simulink model "ex11"  (Simulink 6.0)
settings: Solver=VariableStepDiscrete  StartTime=0.0  StopTime=2  RelTol=1e-3
libraries: commutil2 x4, commsink2 x2, commdigbbndam2 x2, commfilt2 x2, dspsigops x2, commchan2 x1, commrandsrc2 x1
settings Model: LastModifiedBy=lxy

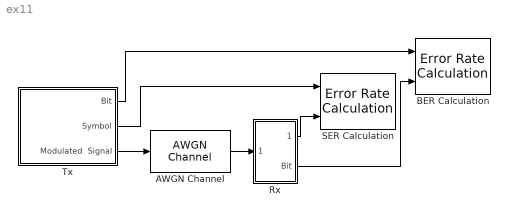
== system ex11 ==
  AWGN Channel : commchan2/AWGN Channel  seed=1234  noiseMode="Signal to noise ratio  (Es/No)"  EbNodB=10  EsNodB=SNR  SNRdB=10  bitsPerSym=1  Ps=0.5  Tsym=1/100000  variance=1
  BER Calculation : commsink2/Error Rate Calculation  N=0  st_delay=16  cp_mode=Entire frame  subframe=[]  PMode=Workspace  WsName=BER  RsMode2=off  stop=off  numErr=100  maxBits=1e6
  Rx : Subsystem
  SER Calculation : commsink2/Error Rate Calculation  N=0  st_delay=8  cp_mode=Entire frame  subframe=[]  PMode=Workspace  WsName=SER  RsMode2=off  stop=off  numErr=100  maxBits=1e6
  Tx : Subsystem
  wires:
  Tx/3(Modulated  Signal) -> AWGN Channel/1
  AWGN Channel/1 -> Rx/1(In1)
  Tx/2(Symbol) -> SER Calculation/1
  Rx/1(Symbol) -> SER Calculation/2
  Tx/1(Bit) -> BER Calculation/1
  Rx/2(Bit) -> BER Calculation/2

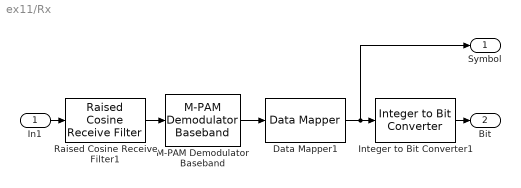
== system ex11/Rx ==
  In1 : Inport  Port=1  LatchInput=off
  Data Mapper1 : commutil2/Data Mapper  MapMode=Gray to Binary  M=4  MapVec=[0 1 3 2 7 6 4 5]
  Integer to Bit Converter1 : commutil2/Integer to Bit Converter  nbits=2
  M-PAM Demodulator Baseband : commdigbbndam2/M-PAM Demodulator Baseband  M=4  OutType=Integer  Dec=Binary  PowType=Min. distance between symbols  MinDist=2  AvgPow=1  PeakPow=1  numSamp=1
  Raised Cosine Receive Filter1 : commfilt2/Raised Cosine Receive Filter  filtType=Square root  N=10  D=4  R=0.25  sampMode=Frame-based  rateMode=Downsampling  downFactor=10  downOffset=0  checkGain=Normalized  filterGain=1  checkCoeff=off  variableName=rcRxFilt1  launchFVT=off
  Symbol : Outport
  Bit : Outport  Port=2
  wires:
  M-PAM Demodulator Baseband/1 -> Data Mapper1/1
  Integer to Bit Converter1/1 -> Bit/1
  Data Mapper1/1 -> Integer to Bit Converter1/1, Symbol/1
  In1/1 -> Raised Cosine Receive Filter1/1
  Raised Cosine Receive Filter1/1 -> M-PAM Demodulator Baseband/1

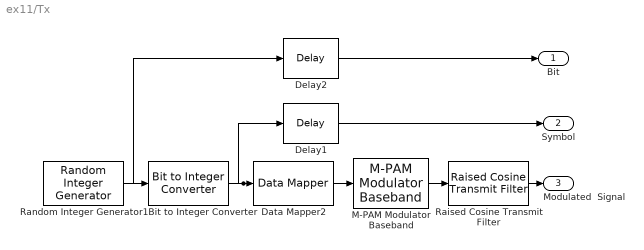
== system ex11/Tx ==
  Bit to Integer Converter : commutil2/Bit to Integer Converter  nbits=2
  Data Mapper2 : commutil2/Data Mapper  MapMode=Binary to Gray  M=4  MapVec=[0 1 3 2 7 6 4 5]
  Delay1 : dspsigops/Delay  dly_unit=Samples  delay=8  ic_detail=off  dif_ic_for_ch=off  dif_ic_for_dly=off  ic=0  reset_popup=None
  Delay2 : dspsigops/Delay  dly_unit=Samples  delay=16  ic_detail=off  dif_ic_for_ch=off  dif_ic_for_dly=off  ic=0  reset_popup=None
  M-PAM Modulator Baseband : commdigbbndam2/M-PAM Modulator Baseband  M=4  InType=Integer  Enc=Binary  PowType=Min. distance between symbols  MinDist=2  AvgPow=1  PeakPow=1  numSamp=1
  Raised Cosine Transmit Filter : commfilt2/Raised Cosine Transmit Filter  filtType=Square root  D=4  R=0.25  sampMode=Frame-based  N=10  checkGain=Normalized  filterGain=1  checkCoeff=off  variableName=rcTxFilt  launchFVT=off
  Random Integer Generator1 : commrandsrc2/Random Integer Generator  mul=2  seed=37  Ts=1/200000  frameBased=on  sampPerFrame=200000  orient=off
  Bit : Outport
  Symbol : Outport  Port=2
  Modulated  Signal : Outport  Port=3
  wires:
  M-PAM Modulator Baseband/1 -> Raised Cosine Transmit Filter/1
  Data Mapper2/1 -> M-PAM Modulator Baseband/1
  Bit to Integer Converter/1 -> Data Mapper2/1, Delay1/1
  Random Integer Generator1/1 -> Bit to Integer Converter/1, Delay2/1
  Raised Cosine Transmit Filter/1 -> Modulated  Signal/1
  Delay1/1 -> Symbol/1
  Delay2/1 -> Bit/1
